simulink model "state_feedback_controller"  (R2018a)
settings: Solver=VariableStepAuto  StartTime=0.0  StopTime=10.0  FixedStep=1e-6  RelTol=1e-3
undefined symbols (not defined in the file): K, L, M, Ms_den, Ms_num, SquareWave, sys, x0
settings Model: Creator=julio  LastModifiedBy=julio

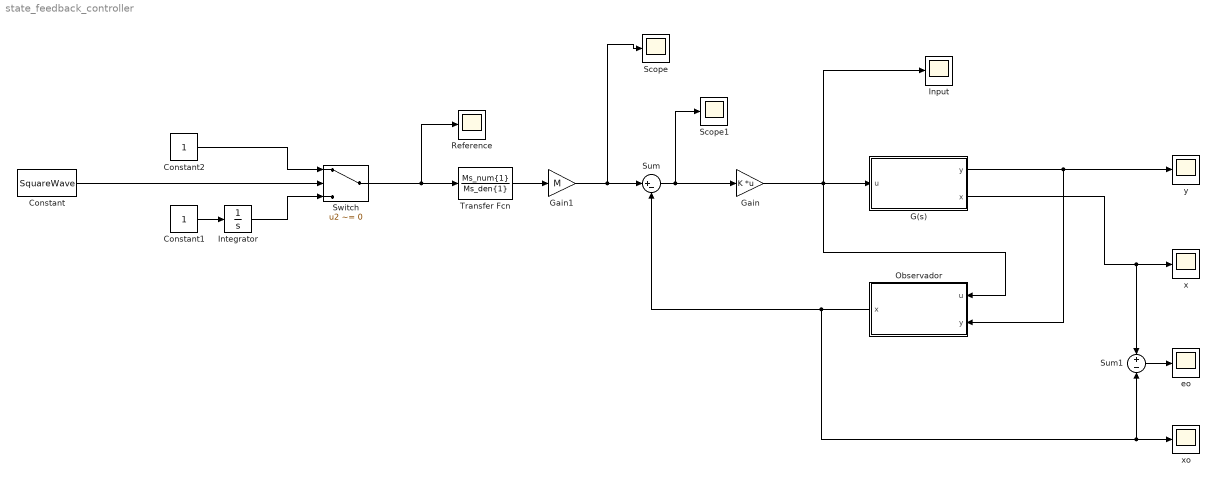
== system state_feedback_controller ==
  Constant : Constant  Value=SquareWave
  Constant1 : Constant
  Constant2 : Constant
  G(s) : Subsystem
  Gain : Gain  Gain=K  Multiplication=Matrix(K*u)
  Gain1 : Gain  Gain=M
  Input : Scope
  Integrator : Integrator
  Observador : Subsystem
  Reference : Scope
  Scope : Scope
  Scope1 : Scope
  Sum : Sum  Inputs=|+-
  Sum1 : Sum  Inputs=+|-
  Switch : Switch  Criteria=u2 ~= 0
  Transfer Fcn : TransferFcn  Numerator=Ms_num{1}  Denominator=Ms_den{1}
  eo : Scope
  x : Scope
  xo : Scope
  y : Scope
  wires:
  Sum/1 -> Scope1/1, Gain/1
  Gain/1 -> Observador/1(u), G(s)/1(u), Input/1
  Switch/1 -> Reference/1, Transfer Fcn/1
  Constant2/1 -> Switch/1
  Integrator/1 -> Switch/3
  Constant/1 -> Switch/2
  Constant1/1 -> Integrator/1
  G(s)/1(y) -> Observador/2(y), y/1
  G(s)/2(x) -> Sum1/1, x/1
  Observador/1(x) -> Sum1/2, xo/1, Sum/2
  Sum1/1 -> eo/1
  Gain1/1 -> Scope/1, Sum/1
  Transfer Fcn/1 -> Gain1/1

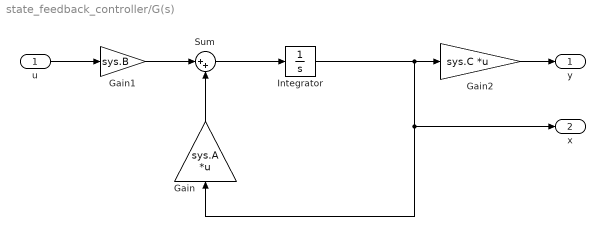
== system state_feedback_controller/G(s) ==
  u : Inport
  Gain : Gain  Gain=sys.A  Multiplication=Matrix(K*u)
  Gain1 : Gain  Gain=sys.B
  Gain2 : Gain  Gain=sys.C  Multiplication=Matrix(K*u)
  Integrator : Integrator  InitialCondition=x0
  Sum : Sum  Inputs=|++
  y : Outport
  x : Outport  Port=2
  wires:
  u/1 -> Gain1/1
  Gain2/1 -> y/1
  Gain1/1 -> Sum/1
  Gain/1 -> Sum/2
  Sum/1 -> Integrator/1
  Integrator/1 -> x/1, Gain/1, Gain2/1

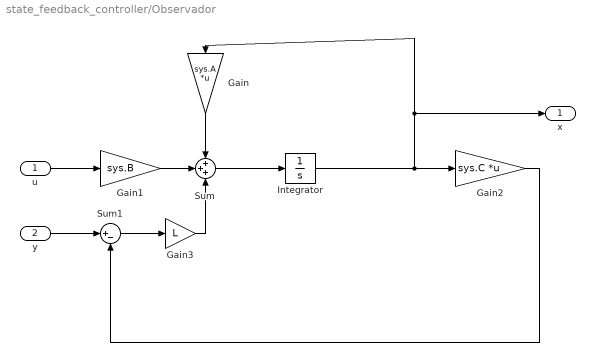
== system state_feedback_controller/Observador ==
  u : Inport
  y : Inport  Port=2
  Gain : Gain  Gain=sys.A  Multiplication=Matrix(K*u)
  Gain1 : Gain  Gain=sys.B
  Gain2 : Gain  Gain=sys.C  Multiplication=Matrix(K*u)
  Gain3 : Gain  Gain=L
  Integrator : Integrator
  Sum : Sum  Inputs=+++
  Sum1 : Sum  Inputs=|+-
  x : Outport
  wires:
  u/1 -> Gain1/1
  Sum/1 -> Integrator/1
  Integrator/1 -> Gain/1, x/1, Gain2/1
  Gain/1 -> Sum/1
  Gain1/1 -> Sum/2
  Gain2/1 -> Sum1/2
  y/1 -> Sum1/1
  Sum1/1 -> Gain3/1
  Gain3/1 -> Sum/3
